simulink model "Mask_Editor"  (R2015b)
settings: Solver=VariableStepAuto  StartTime=0.0  StopTime=10  RelTol=1e-3
StartFcn:
  | open_scope
settings Model: Creator=LUBO  LastModifiedBy=LUBO

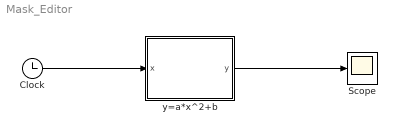
== system Mask_Editor ==
  Clock : Clock
  Scope : Scope
  y=a*x^2+b : Subsystem  mask(Custom){g_a=2, g_b=20}
      mask prompts: g_a "a"; g_b "b"
      mask help: This block supplies a demo of masking.
      mask Help: helpview('xxx.html').
      mask Callback g_a: check_num('g_a');
      mask Callback g_b: check_num('g_b');
      mask Display:
      | %color('red');
      | %text(0,0,'y=a*x^2+b','horizontalAlignment','left','verticalAlignment','bottom');
      | %disp('二次方程');
      | %color('cyan');
      | %text(0.1,0,'hyo','horizontalAlignment','right','verticalAlignment','bottom')
      | a=str2num(get_param(gcbh,'g_a'));
      | b=str2num(get_param(gcbh,'g_b'));
      | t=0:0.1:10;
      | plot(t,a*t.^2+b);
      | %port_label('input',1,'In\spadesuit','texmode','on');
      | %port_label('output',1,'Out\heartsuit','texmode','on');
  wires:
  Clock/1 -> y=a*x^2+b/1(x)
  y=a*x^2+b/1(y) -> Scope/1

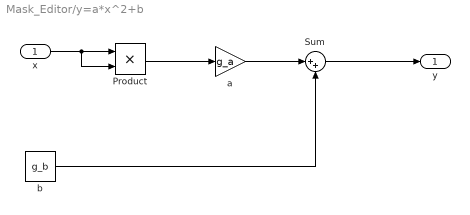
== system Mask_Editor/y=a*x^2+b ==
  x : Inport  Description=x
  Product : Product
  Sum : Sum  Inputs=|++
  a : Gain  Gain=g_a
  b : Constant  Value=g_b
  y : Outport
  wires:
  Product/1 -> a/1
  x/1 -> Product/2, Product/1
  Sum/1 -> y/1
  b/1 -> Sum/2
  a/1 -> Sum/1
